simulink model "CoreComm_Student (2)"  (R2023b)
settings: Solver=FixedStepDiscrete  StartTime=0.0  StopTime=100  FixedStep=SimPara.SysPeriod  RelTol=1e-3
undefined symbols (not defined in the file): SimPara
libraries: commdigbbndpm3 x2, commchan3 x1, commsink2 x1, phaseddetectlib x1, commrandsrc3 x1, commfilt2 x1
settings Model: Creator=paull  LastModifiedBy=bryan
settings SolverCC: AlgebraicLoopSolver=TrustRegion
settings DebuggingCC: UnconnectedInputMsg=warning  UnconnectedOutputMsg=warning  UnconnectedLineMsg=warning
settings ModelReferenceCC: EnableRefExpFcnMdlSchedulingChecks=on
settings SFSimCC: CustomCodeUndefinedFunction=UseInterfaceOnly
settings RTWCC: DLArmComputeVersion=19.05

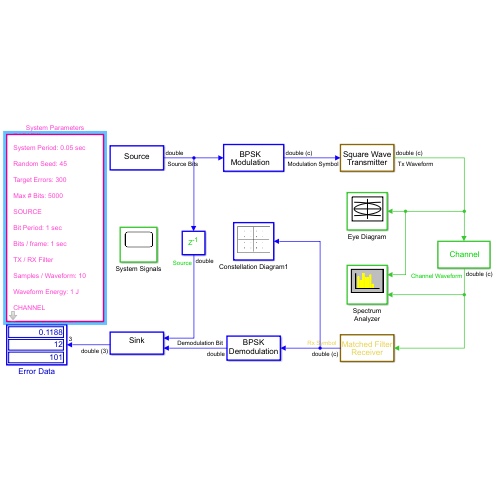
[thumbnail: Simulink's stored preview of the top-level diagram]
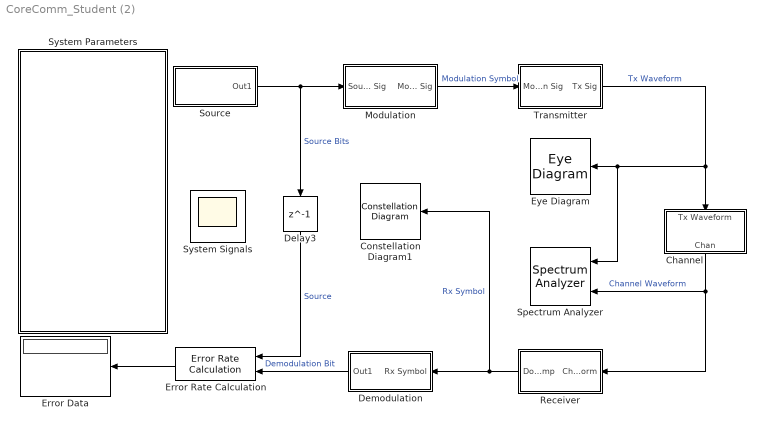
== system CoreComm_Student (2) ==
  Channel : Subsystem
      mask Display: text(40,20,'Channel','horizontalAlignment','center')
  Constellation Diagram1 : ConstellationDiagram  WindowPosition=[29.000000,75.000000,770.000000,662.000000,]  Visible=on  ScopeFrameLocation=window  SymbolsToDisplaySource=Property  SymbolsToDisplay=100  ReferenceConstellation=BPSK  XLimits=[-1.47,1.47]  YLimits=[-1.38,1.38]
  Delay3 : Delay  DelayLength=1  InitialCondition=0
  Demodulation : Subsystem
      mask Display:
      | text(40,20, ...
      |     ['BPSK', ...
      |     '\nDemodulation'], ...
      |     'horizontalAlignment','center')
  Error Data : Display
  Error Rate Calculation : commsink2/Error Rate Calculation  N=0  st_delay=0  cp_mode=Entire frame  subframe=[]  PMode=Port  WsName=ErrorVec  RsMode2=off  stop=on  numErr=SimPara.TargetErr  maxBits=SimPara.MaxNumBits  mask(Error Rate Calculation){}
      mask Display:
      | % This is a new mask on top of the base mask.
      | % Use "View base mask" link below to see the base mask.
      | text(40,20,'Sink','horizontalAlignment','center')
  Eye Diagram : EyeDiagram
  Modulation : Subsystem
      mask Display:
      | text(40,20, ...
      |     ['BPSK', ...
      |     '\nModulation'], ...
      |     'horizontalAlignment','center')
  Receiver : Subsystem
      mask Display:
      | text(40,20, ...
      |     ['Matched Filter', ...
      |     '\nReceiver'], ...
      |     'horizontalAlignment','center')
  Source : Subsystem
      mask Display: text(40,20,'Source','horizontalAlignment','center')
  Spectrum Analyzer : SpectrumAnalyzer  NumInputPorts=2  WindowPosition=[97.000000,43.000000,1440.000000,786.000000,]  Visible=on  ScopeFrameLocation=window  SampleRateSource=Property  SampleRate=SimPara.SampWaveform  FrequencySpan=Start and stop frequencies  StartFrequency=0  StopFrequency=SimPara.SampWaveform/2  AveragingMethod=Exponential  YLimits=[-82.64773538,8.16803679]  ShowLegend=on
      settings: OpenAtSimulationStart=off
  System Parameters : Subsystem  mask{SysPeriod=0.05, RandSeed=45, TargetErr=300, MaxNumBits=5000, BitPeriod=1, BitFrame=1, SampWaveform=10, EnergyWaveform=1, SNR=0}
      mask prompts: SysPeriod "System Period (s)"; RandSeed "Rand. Seed"; TargetErr "Target Errors"; MaxNumBits "Maximum # Bits"; BitPeriod "Bit Period (s)"; BitFrame "Bits / Frame"; SampWaveform "Samples / Waveform"; EnergyWaveform "Waveform Energy (J)"; SNR "Signal-to-Noise (dB)"
      mask init:
      | % Pass the variables to the workspace
      | 
      | info.Mask = gcb;
      | info.SysPeriod=SysPeriod;
      | info.RandSeed = RandSeed;
      | info.TargetErr = TargetErr;
      | info.MaxNumBits = MaxNumBits;
      | info.BitPeriod = BitPeriod;
      | info.BitFrame = BitFrame;
      | info.SampWaveform = SampWaveform;
      | info.EnergyWaveform = EnergyWaveform;
      | info.SNR = SNR;
      | 
      | % Port the mask variables to the base workspace to be accessed by other blocks
      | assignin('base', 'SimPara', info);
      mask DialogControl SysVar Prompt: SYSTEM VARIABLES
      mask DialogControl SourceVar Prompt: SOURCE VARIABLES
      mask DialogControl TxRxFilterVar Prompt: TX/RX FILTER VARIABLES
      mask DialogControl ChanVar Prompt: CHANNEL VARIABLES
      mask Display:
      | text( ...
      |     10, 140, ...
      |     [ ...
      |     'SYSTEM', ...
      |     '\n\nSystem Period: ', num2str(SysPeriod), ' sec', ...
      |     '\n\nRandom Seed: ', num2str(RandSeed), ...
      |     '\n\nTarget Errors: ', num2str(TargetErr), ...
      |     '\n\nMax # Bits: ', num2str(MaxNumBits), ...
      |     '\n\nSOURCE', ...
      |     '\n\nBit Period: ', num2str(BitPeriod), ' sec', ...
      |     '\n\nBits / frame: ', num2str(BitFrame), ' sec', ...
      |     '\n\nTX / RX Filter', ...
      |     '\n\nSamples / Waveform: ', num2str(SampWaveform), ...
      |     '\n\nWaveform Energy: ', num2str(EnergyWaveform), ' J', ...
      |     '\n\nCHANNEL', ...
      |     '\n\nSignal-to-Noise: ', num2str(SNR), ' dB'], ...
      |     'horizontalAlignment', 'left' ...
      |     )
  System Signals : Scope
      settings: Floating=on
  Transmitter : Subsystem
      mask Display:
      | text(40,20, ...
      |     ['Square Wave', ...
      |     '\nTransmitter'], ...
      |     'horizontalAlignment','center')
  wires:
  Error Rate Calculation/1 -> Error Data/1
  Source/1(Out1) -> Delay3/1, Modulation/1(Source Sig)  "Source Bits"
  Modulation/1(Modulation Sig) -> Transmitter/1(Modulation Sig)  "Modulation Symbol"
  Transmitter/1(Tx Sig) -> Spectrum Analyzer/1, Eye Diagram/1, Channel/1(Tx Waveform)  "Tx Waveform"
  Channel/1(Chan) -> Receiver/1(Channel Waveform), Spectrum Analyzer/2  "Channel Waveform"
  Demodulation/1(Out1) -> Error Rate Calculation/2  "Demodulation Bit"
  Receiver/1(Down Samp) -> Constellation Diagram1/1, Demodulation/1(Rx Symbol)  "Rx Symbol"
  Delay3/1 -> Error Rate Calculation/1  "Source"

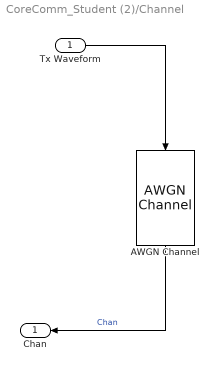
== system CoreComm_Student (2)/Channel ==
  Tx Waveform : Inport
  AWGN Channel : commchan3/AWGN Channel  LegacyMode=on  NoiseMethod="Signal to noise ratio  (SNR)"  noiseMode="Signal to noise ratio  (SNR)"  EbNo=3  EsNo=3  SNR=SimPara.SNR  BitsPerSymbol=1  SignalPower=1  SamplesPerSymbol=1  SymbolPeriod=1/3  VarianceSource=Parameter  Variance=0.5  RandomStream=Global stream  Seed=SimPara.RandSeed  SimulateUsing=Code generation
  Chan : Outport
  wires:
  AWGN Channel/1 -> Chan/1  "Chan"
  Tx Waveform/1 -> AWGN Channel/1

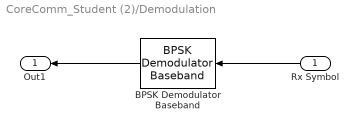
== system CoreComm_Student (2)/Demodulation ==
  Rx Symbol : Inport
  BPSK Demodulator Baseband : commdigbbndpm3/BPSK Demodulator Baseband  DecType=Hard decision  VarSource=Dialog  Variance=1  Ph=0  outDtype=Inherit via internal rule  derotateFactorWordLen=16  derotateFactorDataTypeStr=Inherit: Same word length as input  derotateFactorLastDataTypeStr=Inherit: Same word length as input
  Out1 : Outport
  wires:
  BPSK Demodulator Baseband/1 -> Out1/1
  Rx Symbol/1 -> BPSK Demodulator Baseband/1

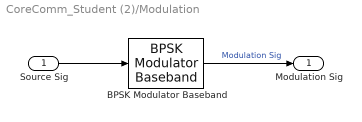
== system CoreComm_Student (2)/Modulation ==
  Source Sig : Inport
  BPSK Modulator Baseband : commdigbbndpm3/BPSK Modulator Baseband  Ph=0  outDtype=double  outWordLen=16  outUDDataType=sfix(16)  outFracLenMode=Best precision  outFracLen=15  outDataTypeStr=double  outLastDataTypeStr=double
  Modulation Sig : Outport
  wires:
  BPSK Modulator Baseband/1 -> Modulation Sig/1  "Modulation Sig"
  Source Sig/1 -> BPSK Modulator Baseband/1

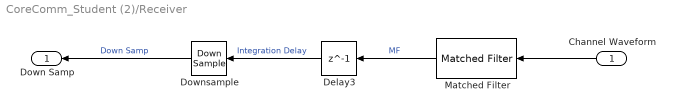
== system CoreComm_Student (2)/Receiver ==
  Channel Waveform : Inport
  Delay3 : Delay  DelayLength=1  InitialCondition=0
  Downsample : DownSample  N=SimPara.SampWaveform  RateOptions=Allow multirate processing
  Matched Filter : phaseddetectlib/Matched Filter  CoefficientsSource=Property  Coefficients=sqrt(1/SimPara.SampWaveform)*ones(SimPara.SampWaveform,1)  SpectrumWindow=None  CustomSpectrumWindow=@hamming  SpectrumRange=[ 0, 1e5 ]  SampleRateFromInputCheckbox=on  SampleRate=1e6  SidelobeAttenuation=30  Beta=0.5  Nbar=4  GainOutputPort=off  MaximumNumInputSamplesSource=Auto  MaximumNumInputSamples=100  SimulateUsing=Interpreted execution
  Down Samp : Outport
  wires:
  Matched Filter/1 -> Delay3/1  "MF"
  Delay3/1 -> Downsample/1  "Integration Delay"
  Channel Waveform/1 -> Matched Filter/1
  Downsample/1 -> Down Samp/1  "Down Samp"

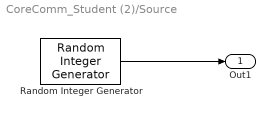
== system CoreComm_Student (2)/Source ==
  Random Integer Generator : commrandsrc3/Random Integer Generator  SetSize=2  SeedSource=Parameter  Seed=SimPara.RandSeed  SampleTime=SimPara.BitPeriod  SamplesPerFrame=SimPara.BitFrame  OutputDataType=double  SimulateUsing=Interpreted execution
  Out1 : Outport
  wires:
  Random Integer Generator/1 -> Out1/1

== system CoreComm_Student (2)/System Parameters ==

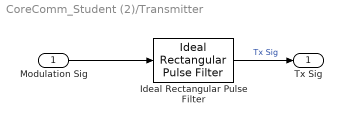
== system CoreComm_Student (2)/Transmitter ==
  Modulation Sig : Inport
  Ideal Rectangular Pulse Filter : commfilt2/Ideal Rectangular Pulse Filter  pulseLen=SimPara.SampWaveform  pulseDelay=0  RateOptions=Allow multirate processing  sampMode=Mute  normCheck=on  normMode=Energy per pulse  filterGain=SimPara.EnergyWaveform  saveAsFlag=0  roundingMode=Floor  overflowMode=off  firstCoeffDataTypeStr=Inherit: Same word length as input  firstCoeffMin=[]  firstCoeffMax=[]  firstCoeffLastDataTypeStr=Inherit: Same word length as input  outputDataTypeStr=Inherit: Same as accumulator  outputMin=[]  outputMax=[]  outputLastDataTypeStr=Inherit: Same as accumulator
  Tx Sig : Outport
  wires:
  Ideal Rectangular Pulse Filter/1 -> Tx Sig/1  "Tx Sig"
  Modulation Sig/1 -> Ideal Rectangular Pulse Filter/1
